simulink model "double_loop"  (R2017a)
settings: Solver=VariableStepAuto  StartTime=0.0  StopTime=30  RelTol=1e-3
libraries: simulink x2
settings Model: Creator=Zichong Lu  LastModifiedBy=Zichong Lu

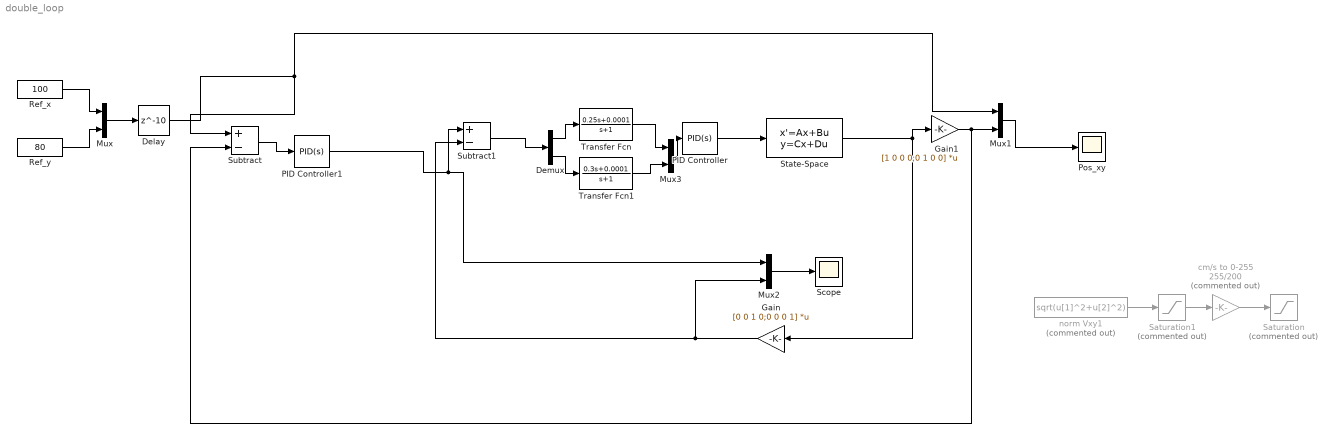
== system double_loop ==
  Delay : Delay  DelayLength=10
  Demux : Demux  Outputs=2
  Gain : Gain  Gain=[0 0 1 0;0 0 0 1]  Multiplication=Matrix(K*u) (u vector)
  Gain1 : Gain  Gain=[1 0 0 0;0 1 0 0]  Multiplication=Matrix(K*u) (u vector)
  Mux{,1..3} (4 alike) : Mux  Inputs=2
  PID Controller : simulink/Continuous/PID Controller  Controller=PID  TimeDomain=Continuous-time  SampleTime=-1  IntegratorMethod=Forward Euler  FilterMethod=Forward Euler  Form=Parallel  UseFilter=on  ControllerParametersSource=internal  P=0.01  I=0  D=0  N=100  InitialConditionSource=internal  InitialConditionForIntegrator=0  InitialConditionForFilter=0  ExternalReset=none  LimitOutput=off  UpperSaturationLimit=inf  LowerSaturationLimit=-inf  LinearizeAsGain=on  AntiWindupMode=none  Kb=1  TrackingMode=off  Kt=1  PParamMin=[]  PParamMax=[]  IParamMin=[]  IParamMax=[]  DParamMin=[]  DParamMax=[]  NParamMin=[]  NParamMax=[]  KbParamMin=[]  KbParamMax=[]  KtParamMin=[]  KtParamMax=[]  POutMin=[]  POutMax=[]  IOutMin=[]  IOutMax=[]  DOutMin=[]  DOutMax=[]  NOutMin=[]  NOutMax=[]  KbOutMin=[]  KbOutMax=[]  KtOutMin=[]  KtOutMax=[]  IntegratorOutMin=[]  IntegratorOutMax=[]  FilterOutMin=[]  FilterOutMax=[]  SumOutMin=[]  SumOutMax=[]  SumI1OutMin=[]  SumI1OutMax=[]  SumI2OutMin=[]  SumI2OutMax=[]  SumI3OutMin=[]  SumI3OutMax=[]  SumDOutMin=[]  SumDOutMax=[]  SaturationOutMin=[]  SaturationOutMax=[]  IntegratorContinuousStateAttributes=''  IntegratorStateMustResolveToSignalObject=off  IntegratorRTWStateStorageClass=Auto  FilterContinuousStateAttributes=''  FilterStateMustResolveToSignalObject=off  FilterRTWStateStorageClass=Auto  DifferentiatorICPrevScaledInput=0  DifferentiatorOutMin=[]  DifferentiatorOutMax=[]  InitialConditionSetting=State (most efficient)
  PID Controller1 : simulink/Continuous/PID Controller  Controller=PID  TimeDomain=Continuous-time  SampleTime=-1  IntegratorMethod=Forward Euler  FilterMethod=Forward Euler  Form=Parallel  UseFilter=on  ControllerParametersSource=internal  P=90  I=0  D=1.5  N=100  InitialConditionSource=internal  InitialConditionForIntegrator=0  InitialConditionForFilter=0  ExternalReset=none  LimitOutput=off  UpperSaturationLimit=inf  LowerSaturationLimit=-inf  LinearizeAsGain=on  AntiWindupMode=none  Kb=1  TrackingMode=off  Kt=1  PParamMin=[]  PParamMax=[]  IParamMin=[]  IParamMax=[]  DParamMin=[]  DParamMax=[]  NParamMin=[]  NParamMax=[]  KbParamMin=[]  KbParamMax=[]  KtParamMin=[]  KtParamMax=[]  POutMin=[]  POutMax=[]  IOutMin=[]  IOutMax=[]  DOutMin=[]  DOutMax=[]  NOutMin=[]  NOutMax=[]  KbOutMin=[]  KbOutMax=[]  KtOutMin=[]  KtOutMax=[]  IntegratorOutMin=[]  IntegratorOutMax=[]  FilterOutMin=[]  FilterOutMax=[]  SumOutMin=[]  SumOutMax=[]  SumI1OutMin=[]  SumI1OutMax=[]  SumI2OutMin=[]  SumI2OutMax=[]  SumI3OutMin=[]  SumI3OutMax=[]  SumDOutMin=[]  SumDOutMax=[]  SaturationOutMin=[]  SaturationOutMax=[]  IntegratorContinuousStateAttributes=''  IntegratorStateMustResolveToSignalObject=off  IntegratorRTWStateStorageClass=Auto  FilterContinuousStateAttributes=''  FilterStateMustResolveToSignalObject=off  FilterRTWStateStorageClass=Auto  DifferentiatorICPrevScaledInput=0  DifferentiatorOutMin=[]  DifferentiatorOutMax=[]  InitialConditionSetting=State (most efficient)
  Pos_xy : Scope
  Ref_x : Constant  Value=100
  Ref_y : Constant  Value=80
  Saturation : Saturate  Commented=on  UpperLimit=255  LowerLimit=0
  Saturation1 : Saturate  Commented=on  UpperLimit=20  LowerLimit=-20
  Scope : Scope
  State-Space : StateSpace  A=[0 0 1 0;0 0 0 1;0 0 0 0;0 0 0 0]  B=[0 0;0 0;2.22 0;0 2.22]  C=[1 0 0 0;0 1 0 0;0 0 1 0;0 0 0 1]  D=[0 0;0 0;0 0;0 0]  X0=0
  Subtract : Sum  Inputs=+-
  Subtract1 : Sum  Inputs=+-
  Transfer Fcn : TransferFcn  Numerator=[0.25 0.0001]  Denominator=[1 1]
  Transfer Fcn1 : TransferFcn  Numerator=[0.3 0.0001]  Denominator=[1 1]
  cm/s to 0-255 : Gain  Commented=on  Gain=255/200  SaturateOnIntegerOverflow=on  OutDataTypeStr=Inherit: Same as input  ParamDataTypeStr=Inherit: Same as input
  norm Vxy1 : Fcn  Commented=on  Expr=sqrt(u[1]^2+u[2]^2)
  wires:
  Ref_x/1 -> Mux/1
  Ref_y/1 -> Mux/2
  Mux1/1 -> Pos_xy/1
  PID Controller/1 -> State-Space/1
  norm Vxy1/1 -> Saturation1/1
  Saturation1/1 -> cm/s to 0-255/1
  cm/s to 0-255/1 -> Saturation/1
  State-Space/1 -> Gain1/1, Gain/1
  PID Controller1/1 -> Mux2/1, Subtract1/1
  Mux2/1 -> Scope/1
  Gain/1 -> Mux2/2, Subtract1/2
  Gain1/1 -> Subtract/2, Mux1/2
  Subtract/1 -> PID Controller1/1
  Mux/1 -> Delay/1
  Demux/2 -> Transfer Fcn1/1
  Demux/1 -> Transfer Fcn/1
  Transfer Fcn/1 -> Mux3/1
  Transfer Fcn1/1 -> Mux3/2
  Mux3/1 -> PID Controller/1
  Delay/1 -> Mux1/1, Subtract/1
  Subtract1/1 -> Demux/1
